simulink model "FOC_Modified"  (R2016b)
settings: Solver=FixedStepDiscrete  StartTime=0.0  StopTime=10.0  RelTol=1e-3  EnableMultiTasking=on
PreLoadFcn:
  | hdlcoderFocCurrentFixptHdlData
undefined symbols (not defined in the file): dataRange, paramCurrentControlSatVoltage
libraries: simulink x3
settings Model: Creator=mcorless  LastModifiedBy=paul.rogers
settings DataIOCC: LimitDataPoints=on  SaveFormat=Array
settings OptimizationCC: BlockReduction=off  ConditionallyExecuteInputs=off  DefaultParameterBehavior=Inlined  InlineInvariantSignals=on  LifeSpan=1
settings DebuggingCC: ArtificialAlgebraicLoopMsg=error  SolverPrmCheckMsg=warning  InheritedTsInSrcMsg=none  SingleTaskRateTransMsg=error  ParameterPrecisionLossMsg=none  SFUnexpectedBacktrackingDiag=warning  SFNoUnconditionalDefaultTransitionDiag=warning  SFExecutionAtInitializationDiag=none
settings HardwareCC: ProdBitPerPointer=32  ProdBitPerSizeT=32  ProdBitPerPtrDiffT=32  ProdLargestAtomicFloat=None  ProdIntDivRoundTo=Undefined  ProdEndianess=Unspecified  ProdWordSize=32  ProdHWDeviceType=ASIC/FPGA  ProdEqTarget=off
settings ModelReferenceCC: PropagateSignalLabelsOutOfModel=off
settings GRTTargetCC: TargetLangStandard=C89/C90 (ANSI)  GeneratePreprocessorConditionals=Disable all
settings ConfigComp: CovMetricSettings=dw  CovHtmlReporting=on  CovSaveCumulativeToWorkspaceVar=on  CovSaveSingleToWorkspaceVar=on  CovExternalEMLEnable=off  CovSFcnEnable=off

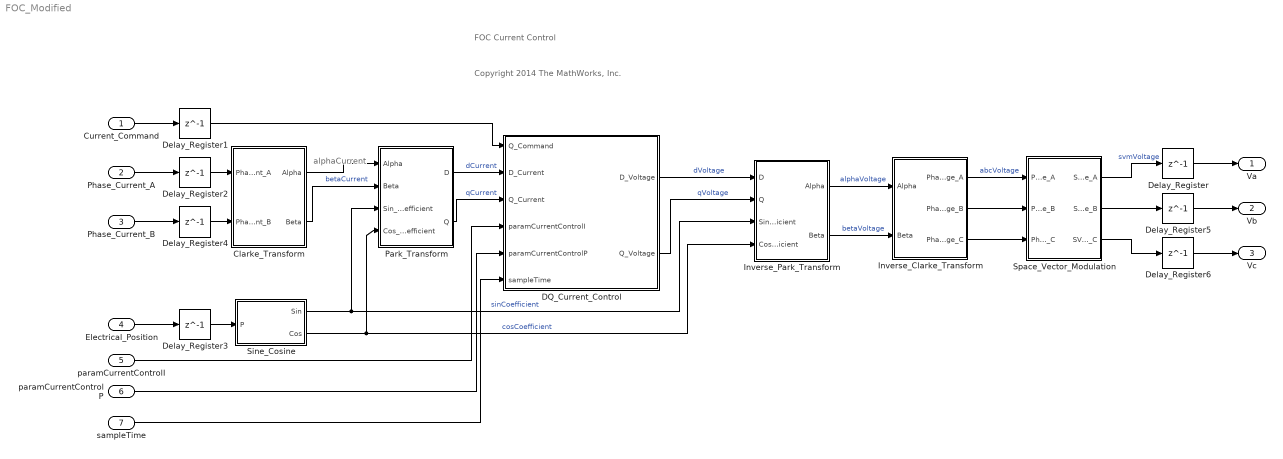
== system FOC_Modified ==
  note: alphaCurrent
  note: FOC Current Control
  note: Copyright 2014 The MathWorks, Inc.
  Current_Command : Inport  OutMin=dataRange.PhaseCurrent.Min  OutMax=dataRange.PhaseCurrent.Max  OutDataTypeStr=fixdt(1,16,12)  SampleTime=0.000000081
  Phase_Current_A : Inport  Port=2  OutMin=dataRange.PhaseCurrent.Min  OutMax=dataRange.PhaseCurrent.Max  OutDataTypeStr=fixdt(1,16,12)  SampleTime=0.000000081
  Phase_Current_B : Inport  Port=3  OutMin=dataRange.PhaseCurrent.Min  OutMax=dataRange.PhaseCurrent.Max  OutDataTypeStr=fixdt(1,16,12)  SampleTime=0.000000081
  Electrical_Position : Inport  Port=4  OutMin=0  OutMax=2*pi  OutDataTypeStr=fixdt(1,16,12)  SampleTime=0.000000081
  paramCurrentControlI : Inport  Port=5  OutDataTypeStr=fixdt(1,16,3)  SampleTime=0.000000081
  paramCurrentControlP : Inport  Port=6  OutDataTypeStr=fixdt(1,16,8)  SampleTime=0.000000081
  sampleTime : Inport  Port=7  OutDataTypeStr=fixdt(1,16,30)  SampleTime=0.000000081
  Clarke_Transform : Subsystem
      mask Display:
      | port_label('input',1,'ABC')
      | port_label('output',1,'\alpha','texmode', 'on')
      | port_label('output',2,'\beta','texmode', 'on')
  DQ_Current_Control : Subsystem
  Delay_Register{,1..6} (7 alike) : Delay  DelayLength=1
  Inverse_Clarke_Transform : Subsystem  VariantControl=INVERSE_CLARKE_TRANSFORM
      mask Display:
      | port_label('input',1,'\alpha','texmode', 'on')
      | port_label('input',2,'\beta','texmode', 'on')
      | port_label('output',1,'ABC')
  Inverse_Park_Transform : Subsystem
      mask Display:
      | port_label('input',1,'D')
      | port_label('input',2,'Q')
      | port_label('input',3,'Sin')
      | port_label('input',4,'Cos')
      | port_label('output',1,'\alpha','texmode', 'on')
      | port_label('output',2,'\beta','texmode', 'on')
  Park_Transform : Subsystem
      mask Display:
      | port_label('input',1,'\alpha','texmode', 'on')
      | port_label('input',2,'\beta','texmode', 'on')
      | port_label('input',3,'Sin')
      | port_label('input',4,'Cos')
      | port_label('output',1,'D')
      | port_label('output',2,'Q')
  Sine_Cosine : Subsystem
  Space_Vector_Modulation : Subsystem  VariantControl=SpaceVectorModulation_JB
      mask Display:
      | plot([0.000 0.020 0.041 0.061 0.082 0.102 0.122 0.143 0.163 0.184 0.204 0.224 0.245 0.265 0.286 0.306 0.327 0.347 0.367 0.388 0.408 0.429 0.449 0.469 0.490 0.510 0.531 0.551 0.571 0.592 0.612 0.633 0.653 0.673 0.694 0.714 0.735 0.755 0.776 0.796 0.816 0.837 0.857 0.878 0.898 0.918 0.939 0.959 0.980 1.000 ], ...
      |      [0.500 0.586 0.671 0.753 0.831 0.858 0.875 0.885 0.890 0.887 0.879 0.864 0.844 0.855 0.872 0.884 0.889 0.888 0.881 0.867 0.847 0.793 0.713 0.629 0.543 0.457 0.371 0.287 0.207 0.153 0.133 0.119 0.112 0.111 0.116 0.128 0.145 0.156 0.136 0.121 0.113 0.110 0.115 0.125 0.142 0.169 0.247 0.329 0.414 0.500 ])
  Va : Outport
  Vb : Outport  Port=2
  Vc : Outport  Port=3
  wires:
  Sine_Cosine/1(Sin) -> Park_Transform/3(Sin_Coefficient), Inverse_Park_Transform/3(Sin_Coefficient)  "sinCoefficient"
  Sine_Cosine/2(Cos) -> Park_Transform/4(Cos_Coefficient), Inverse_Park_Transform/4(Cos_Coefficient)  "cosCoefficient"
  Inverse_Clarke_Transform/1(Phase_Voltage_A) -> Space_Vector_Modulation/1(Phase_Voltage_A)  "abcVoltage"
  Electrical_Position/1 -> Delay_Register3/1
  Phase_Current_A/1 -> Delay_Register2/1
  Clarke_Transform/1(Alpha) -> Park_Transform/1(Alpha)
  Clarke_Transform/2(Beta) -> Park_Transform/2(Beta)  "betaCurrent"
  Inverse_Park_Transform/1(Alpha) -> Inverse_Clarke_Transform/1(Alpha)  "alphaVoltage"
  Inverse_Park_Transform/2(Beta) -> Inverse_Clarke_Transform/2(Beta)  "betaVoltage"
  Park_Transform/1(D) -> DQ_Current_Control/2(D_Current)  "dCurrent"
  Park_Transform/2(Q) -> DQ_Current_Control/3(Q_Current)  "qCurrent"
  Current_Command/1 -> Delay_Register1/1
  DQ_Current_Control/1(D_Voltage) -> Inverse_Park_Transform/1(D)  "dVoltage"
  DQ_Current_Control/2(Q_Voltage) -> Inverse_Park_Transform/2(Q)  "qVoltage"
  Delay_Register1/1 -> DQ_Current_Control/1(Q_Command)
  Delay_Register2/1 -> Clarke_Transform/1(Phase_Current_A)
  Delay_Register3/1 -> Sine_Cosine/1(P)
  paramCurrentControlI/1 -> DQ_Current_Control/4(paramCurrentControlI)
  paramCurrentControlP/1 -> DQ_Current_Control/5(paramCurrentControlP)
  sampleTime/1 -> DQ_Current_Control/6(sampleTime)
  Phase_Current_B/1 -> Delay_Register4/1
  Delay_Register4/1 -> Clarke_Transform/2(Phase_Current_B)
  Inverse_Clarke_Transform/2(Phase_Voltage_B) -> Space_Vector_Modulation/2(Phase_Voltage_B)
  Inverse_Clarke_Transform/3(Phase_Voltage_C) -> Space_Vector_Modulation/3(Phase_Voltage_C)
  Space_Vector_Modulation/2(SVM_Phase_Voltage_B) -> Delay_Register5/1
  Space_Vector_Modulation/1(SVM_Phase_Voltage_A) -> Delay_Register/1  "svmVoltage"
  Space_Vector_Modulation/3(SVM_Phase_Voltage_C) -> Delay_Register6/1
  Delay_Register5/1 -> Vb/1
  Delay_Register6/1 -> Vc/1
  Delay_Register/1 -> Va/1

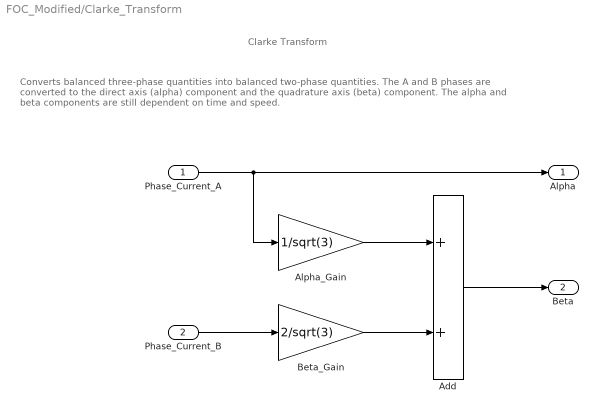
== system FOC_Modified/Clarke_Transform ==
  note: Clarke Transform
  note: Converts balanced three-phase quantities into balanced two-phase quantities.
      | The A and B phases are converted to the direct axis (alpha) component and the quadrature axis (beta) component.
      | The alpha and beta components are still dependent on time and speed.
  Phase_Current_A : Inport
  Phase_Current_B : Inport  Port=2
  Add : Sum  OutDataTypeStr=fixdt(1,16,11)
  Alpha_Gain : Gain  Gain=1/sqrt(3)  ParamDataTypeStr=fixdt(1,16,15)  OutDataTypeStr=fixdt(1,32,29)
  Beta_Gain : Gain  Gain=2/sqrt(3)  ParamDataTypeStr=fixdt(1,16,14)  OutDataTypeStr=fixdt(1,32,28)
  Alpha : Outport
  Beta : Outport  Port=2
  wires:
  Add/1 -> Beta/1
  Phase_Current_B/1 -> Beta_Gain/1
  Beta_Gain/1 -> Add/2
  Alpha_Gain/1 -> Add/1
  Phase_Current_A/1 -> Alpha_Gain/1, Alpha/1

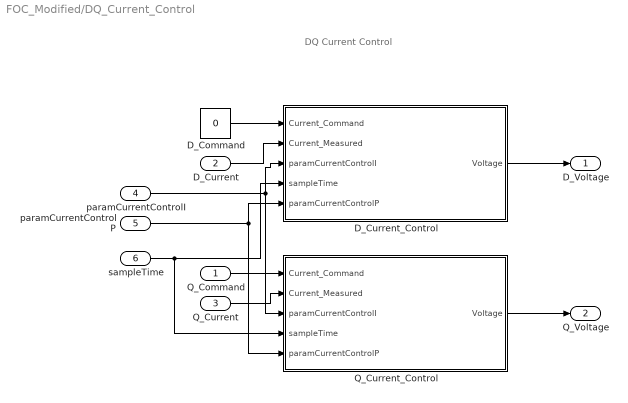
== system FOC_Modified/DQ_Current_Control ==
  note: DQ Current Control
  Q_Command : Inport  SampleTime=0.000000081
  D_Current : Inport  Port=2
  Q_Current : Inport  Port=3
  paramCurrentControlI : Inport  Port=4  SampleTime=0.000000081
  paramCurrentControlP : Inport  Port=5
  sampleTime : Inport  Port=6  SampleTime=0.000000081
  D_Command : Constant  Value=0  OutDataTypeStr=fixdt(1,16,12)  SampleTime=0.000000081
  D_Current_Control : Subsystem  TreatAsAtomicUnit=on
  Q_Current_Control : Subsystem  TreatAsAtomicUnit=on
  D_Voltage : Outport
  Q_Voltage : Outport  Port=2
  wires:
  Q_Current_Control/1(Voltage) -> Q_Voltage/1
  D_Current_Control/1(Voltage) -> D_Voltage/1
  D_Command/1 -> D_Current_Control/1(Current_Command)
  Q_Command/1 -> Q_Current_Control/1(Current_Command)
  Q_Current/1 -> Q_Current_Control/2(Current_Measured)
  D_Current/1 -> D_Current_Control/2(Current_Measured)
  sampleTime/1 -> D_Current_Control/4(sampleTime), Q_Current_Control/4(sampleTime)
  paramCurrentControlI/1 -> D_Current_Control/3(paramCurrentControlI), Q_Current_Control/3(paramCurrentControlI)
  paramCurrentControlP/1 -> D_Current_Control/5(paramCurrentControlP), Q_Current_Control/5(paramCurrentControlP)

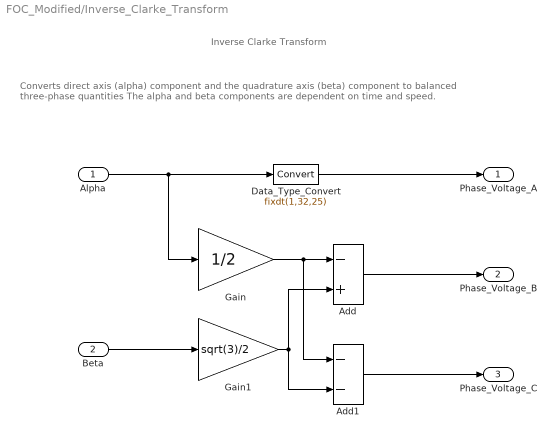
== system FOC_Modified/Inverse_Clarke_Transform ==
  note: Inverse Clarke Transform
  note: Converts direct axis (alpha) component and the quadrature axis (beta) component to balanced three-phase quantities
      | The alpha and beta components are dependent on time and speed.
  Alpha : Inport
  Beta : Inport  Port=2
  Add : Sum  Inputs=-+  OutDataTypeStr=fixdt(1,32,25)
  Add1 : Sum  Inputs=--  OutDataTypeStr=fixdt(1,32,25)
  Data_Type_Convert : DataTypeConversion  OutDataTypeStr=fixdt(1,32,25)  RndMeth=Simplest
  Gain : Gain  Gain=1/2  ParamDataTypeStr=fixdt(1,16,15)  OutDataTypeStr=fixdt(1,32,27)
  Gain1 : Gain  Gain=sqrt(3)/2  ParamDataTypeStr=fixdt(1,16,15)  OutDataTypeStr=fixdt(1,32,26)
  Phase_Voltage_A : Outport
  Phase_Voltage_B : Outport  Port=2
  Phase_Voltage_C : Outport  Port=3
  wires:
  Gain/1 -> Add1/1, Add/1
  Gain1/1 -> Add1/2, Add/2
  Add/1 -> Phase_Voltage_B/1
  Add1/1 -> Phase_Voltage_C/1
  Beta/1 -> Gain1/1
  Alpha/1 -> Gain/1, Data_Type_Convert/1
  Data_Type_Convert/1 -> Phase_Voltage_A/1

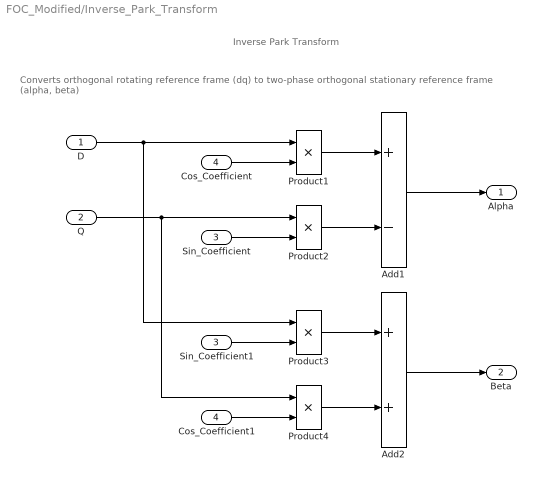
== system FOC_Modified/Inverse_Park_Transform ==
  note: Inverse Park Transform
  note: Converts orthogonal rotating reference frame (dq) to two-phase orthogonal stationary reference frame (alpha, beta)
  D : Inport
  Q : Inport  Port=2
  Sin_Coefficient : Inport  Port=3
  Cos_Coefficient : Inport  Port=4
  Add1 : Sum  Inputs=+-  OutDataTypeStr=fixdt(1,16,10)
  Add2 : Sum  OutDataTypeStr=fixdt(1,16,10)
  Cos_Coefficient1 : InportShadow  Port=4
  Product{1..4} (4 alike) : Product  OutDataTypeStr=fixdt(1,32,27)  RndMeth=Simplest
  Sin_Coefficient1 : InportShadow  Port=3
  Alpha : Outport
  Beta : Outport  Port=2
  wires:
  Add2/1 -> Beta/1
  Add1/1 -> Alpha/1
  Product3/1 -> Add2/1
  Product4/1 -> Add2/2
  Product1/1 -> Add1/1
  Product2/1 -> Add1/2
  Cos_Coefficient1/1 -> Product4/2
  Sin_Coefficient/1 -> Product2/2
  D/1 -> Product3/1, Product1/1
  Q/1 -> Product2/1, Product4/1
  Sin_Coefficient1/1 -> Product3/2
  Cos_Coefficient/1 -> Product1/2

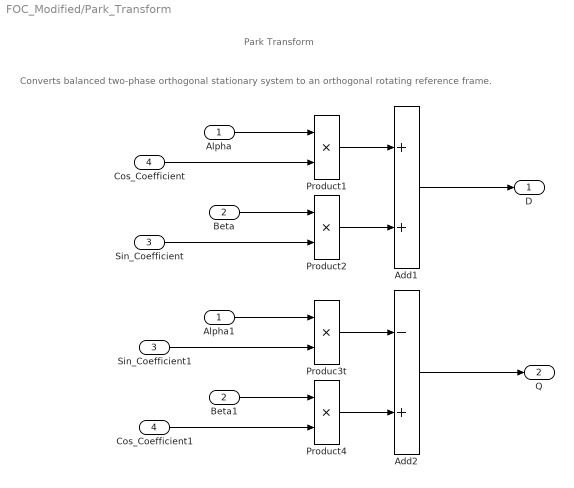
== system FOC_Modified/Park_Transform ==
  note: Park Transform
  note: Converts balanced two-phase orthogonal stationary system to an orthogonal rotating reference frame.
  Alpha : Inport
  Beta : Inport  Port=2
  Sin_Coefficient : Inport  Port=3
  Cos_Coefficient : Inport  Port=4
  Add1 : Sum  OutDataTypeStr=fixdt(1,32,27)
  Add2 : Sum  Inputs=-+  OutDataTypeStr=fixdt(1,32,27)
  Alpha1 : InportShadow
  Beta1 : InportShadow  Port=2
  Cos_Coefficient1 : InportShadow  Port=4
  Produc3t : Product  OutDataTypeStr=fixdt(1,32,28)  RndMeth=Simplest
  Product1 : Product  OutDataTypeStr=fixdt(1,32,28)  RndMeth=Simplest
  Product2 : Product  OutDataTypeStr=fixdt(1,32,27)  RndMeth=Simplest
  Product4 : Product  OutDataTypeStr=fixdt(1,32,27)  RndMeth=Simplest
  Sin_Coefficient1 : InportShadow  Port=3
  D : Outport
  Q : Outport  Port=2
  wires:
  Produc3t/1 -> Add2/1
  Product4/1 -> Add2/2
  Product1/1 -> Add1/1
  Product2/1 -> Add1/2
  Alpha1/1 -> Produc3t/1
  Sin_Coefficient1/1 -> Produc3t/2
  Cos_Coefficient1/1 -> Product4/2
  Beta1/1 -> Product4/1
  Alpha/1 -> Product1/1
  Cos_Coefficient/1 -> Product1/2
  Beta/1 -> Product2/1
  Sin_Coefficient/1 -> Product2/2
  Add1/1 -> D/1
  Add2/1 -> Q/1

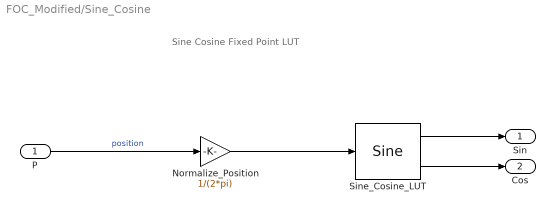
== system FOC_Modified/Sine_Cosine ==
  note: Sine Cosine Fixed Point LUT
  P : Inport
  Normalize_Position : Gain  Gain=1/(2*pi)  ParamDataTypeStr=fixdt(1,16,17)  OutMin=0  OutMax=1  OutDataTypeStr=fixdt(1,32,30)
      settings: AttributesFormatString=|
      | ------------------------------
      | Gain = %<Gain>
  Sine_Cosine_LUT : simulink/Lookup Tables/Sine  Formula=sin(2*pi*u) and cos(2*pi*u)  NumDataPoints=(2^5)+1  OutputWordLength=16  InternalRulePriority=Speed
  Sin : Outport
  Cos : Outport  Port=2
  wires:
  Sine_Cosine_LUT/2 -> Cos/1
  Sine_Cosine_LUT/1 -> Sin/1
  Normalize_Position/1 -> Sine_Cosine_LUT/1
  P/1 -> Normalize_Position/1  "position"

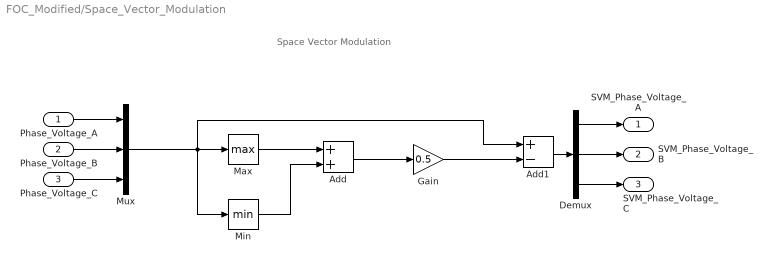
== system FOC_Modified/Space_Vector_Modulation ==
  note: Space Vector Modulation
  Phase_Voltage_A : Inport
  Phase_Voltage_B : Inport  Port=2
  Phase_Voltage_C : Inport  Port=3
  Add : Sum  OutDataTypeStr=fixdt(1,16,8)
  Add1 : Sum  Inputs=+-  OutDataTypeStr=fixdt(1,16,8)
  Demux : Demux  Outputs=3
  Gain : Gain  Gain=0.5  ParamDataTypeStr=fixdt(1,16,15)  OutDataTypeStr=fixdt(1,32,25)
  Max : MinMax  Function=max
  Min : MinMax
  Mux : Mux  Inputs=3
  SVM_Phase_Voltage_A : Outport
  SVM_Phase_Voltage_B : Outport  Port=2
  SVM_Phase_Voltage_C : Outport  Port=3
  wires:
  Add/1 -> Gain/1
  Max/1 -> Add/1
  Min/1 -> Add/2
  Gain/1 -> Add1/2
  Phase_Voltage_C/1 -> Mux/3
  Phase_Voltage_B/1 -> Mux/2
  Phase_Voltage_A/1 -> Mux/1
  Mux/1 -> Add1/1, Min/1, Max/1
  Add1/1 -> Demux/1
  Demux/3 -> SVM_Phase_Voltage_C/1
  Demux/2 -> SVM_Phase_Voltage_B/1
  Demux/1 -> SVM_Phase_Voltage_A/1

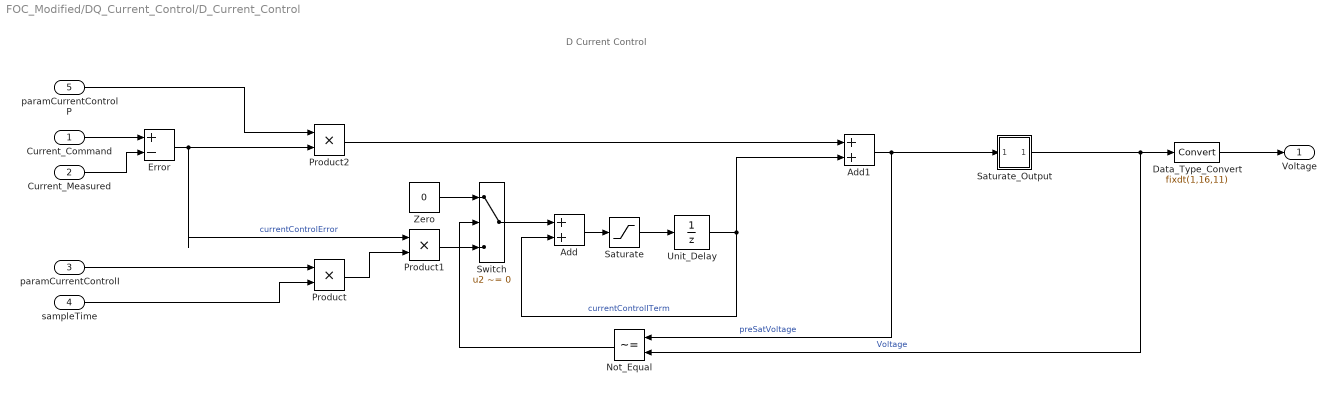
== system FOC_Modified/DQ_Current_Control/D_Current_Control ==
  note: D Current Control
  Current_Command : Inport
  Current_Measured : Inport  Port=2
  paramCurrentControlI : Inport  Port=3
  sampleTime : Inport  Port=4
  paramCurrentControlP : Inport  Port=5
  Add : Sum  OutDataTypeStr=fixdt(1,32,27)
  Add1 : Sum  OutDataTypeStr=fixdt(1,32,20)
  Data_Type_Convert : DataTypeConversion  OutDataTypeStr=fixdt(1,16,11)  RndMeth=Simplest
  Error : Sum  Inputs=+-  OutDataTypeStr=fixdt(1,16,11)
  Not_Equal : RelationalOperator  Operator=~=  OutDataTypeStr=boolean  RndMeth=Nearest
  Product : Product  OutDataTypeStr=fixdt(1,16,19)
  Product1 : Product  OutDataTypeStr=fixdt(1,32,31)
  Product2 : Product
  Saturate : Saturate  UpperLimit=dataRange.DqVoltage.Max  LowerLimit=dataRange.DqVoltage.Min
      settings: AttributesFormatString=|
      | --------------------------------------------
      | Upper = %<UpperLimit>
      | Lower = %<LowerLimit>
  Saturate_Output : Subsystem  mask(Saturate Magnitude){magnitudeLimit=paramCurrentControlSatVoltage}
      mask prompts: magnitudeLimit "Magnitude limit:"
      mask help:
      | Saturates input where:
      |    Upper limit =   Magnitude limit
      |    Lower limit = - Magnitude limit
      settings: AttributesFormatString=|
      | --------------------------------------------
      | Upper limit = %<magnitudeLimit>
      | Lower limit = -%<magnitudeLimit>
      mask Display: plot([0.15 0.85],[.5 .5],[.5 .5],[0.05 0.95],0.15+0.7*[0 .25 .75 1],0.05+0.9*[.25 .25 .75 .75]);
  Switch : Switch  Criteria=u2 ~= 0  OutDataTypeStr=fixdt(1,32,31)
  Unit_Delay : UnitDelay  SampleTime=-1
  Zero : Constant  Value=0  OutDataTypeStr=fixdt(1,16,0)  SampleTime=0.000000081
  Voltage : Outport
  wires:
  Data_Type_Convert/1 -> Voltage/1
  Product1/1 -> Switch/3
  Product/1 -> Product1/2
  sampleTime/1 -> Product/2
  paramCurrentControlI/1 -> Product/1
  Saturate/1 -> Unit_Delay/1
  Zero/1 -> Switch/1
  Switch/1 -> Add/1
  Not_Equal/1 -> Switch/2
  Add/1 -> Saturate/1
  Saturate_Output/1(Out) -> Data_Type_Convert/1, Not_Equal/2  "Voltage"
  Error/1 -> Product2/2, Product1/1  "currentControlError"
  Current_Command/1 -> Error/1
  Add1/1 -> Saturate_Output/1(In), Not_Equal/1  "preSatVoltage"
  Unit_Delay/1 -> Add1/2, Add/2  "currentControlITerm"
  Current_Measured/1 -> Error/2
  Product2/1 -> Add1/1
  paramCurrentControlP/1 -> Product2/1

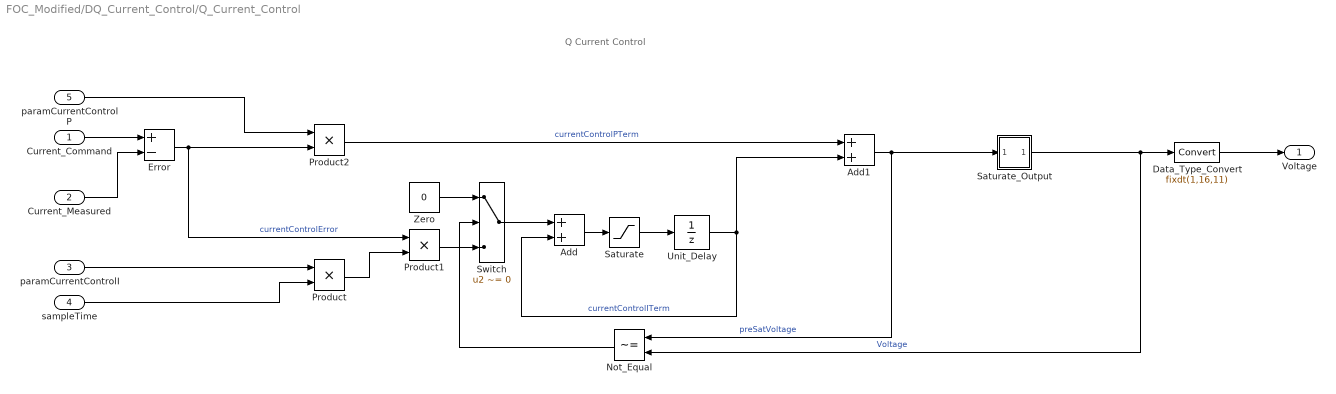
== system FOC_Modified/DQ_Current_Control/Q_Current_Control ==
  note: Q Current Control
  Current_Command : Inport
  Current_Measured : Inport  Port=2
  paramCurrentControlI : Inport  Port=3
  sampleTime : Inport  Port=4
  paramCurrentControlP : Inport  Port=5
  Add : Sum  OutDataTypeStr=fixdt(1,32,27)
  Add1 : Sum  OutDataTypeStr=fixdt(1,32,20)
  Data_Type_Convert : DataTypeConversion  OutDataTypeStr=fixdt(1,16,11)  RndMeth=Simplest
  Error : Sum  Inputs=+-  OutDataTypeStr=fixdt(1,16,11)
  Not_Equal : RelationalOperator  Operator=~=  OutDataTypeStr=boolean  RndMeth=Nearest
  Product : Product  OutDataTypeStr=fixdt(1,16,19)
  Product1 : Product  OutDataTypeStr=fixdt(1,32,31)
  Product2 : Product
  Saturate : Saturate  UpperLimit=dataRange.DqVoltage.Max  LowerLimit=dataRange.DqVoltage.Min
      settings: AttributesFormatString=|
      | --------------------------------------------
      | Upper = %<UpperLimit>
      | Lower = %<LowerLimit>
  Saturate_Output : Subsystem  mask(Saturate Magnitude){magnitudeLimit=paramCurrentControlSatVoltage}
      mask prompts: magnitudeLimit "Magnitude limit:"
      mask help:
      | Saturates input where:
      |    Upper limit =   Magnitude limit
      |    Lower limit = - Magnitude limit
      settings: AttributesFormatString=|
      | --------------------------------------------
      | Upper limit = %<magnitudeLimit>
      | Lower limit = -%<magnitudeLimit>
      mask Display: plot([0.15 0.85],[.5 .5],[.5 .5],[0.05 0.95],0.15+0.7*[0 .25 .75 1],0.05+0.9*[.25 .25 .75 .75]);
  Switch : Switch  Criteria=u2 ~= 0  OutDataTypeStr=fixdt(1,32,31)
  Unit_Delay : UnitDelay  SampleTime=-1
  Zero : Constant  Value=0  OutDataTypeStr=fixdt(1,16,0)  SampleTime=0.000000081
  Voltage : Outport
  wires:
  Current_Measured/1 -> Error/2
  Unit_Delay/1 -> Add/2, Add1/2  "currentControlITerm"
  Add1/1 -> Not_Equal/1, Saturate_Output/1(In)  "preSatVoltage"
  Current_Command/1 -> Error/1
  Product2/1 -> Add1/1  "currentControlPTerm"
  Error/1 -> Product2/2, Product1/1  "currentControlError"
  Saturate_Output/1(Out) -> Not_Equal/2, Data_Type_Convert/1  "Voltage"
  Add/1 -> Saturate/1
  Not_Equal/1 -> Switch/2
  Switch/1 -> Add/1
  Zero/1 -> Switch/1
  Saturate/1 -> Unit_Delay/1
  paramCurrentControlI/1 -> Product/1
  sampleTime/1 -> Product/2
  Product/1 -> Product1/2
  Product1/1 -> Switch/3
  Data_Type_Convert/1 -> Voltage/1
  paramCurrentControlP/1 -> Product2/1

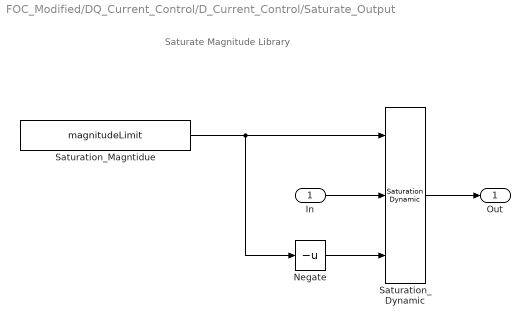
== system FOC_Modified/DQ_Current_Control/D_Current_Control/Saturate_Output ==
  note: Saturate Magnitude Library
  In : Inport
  Negate : UnaryMinus  SampleTime=0.000000081
  Saturation_Dynamic : simulink/Discontinuities/Saturation Dynamic  OutMin=[]  OutMax=[]  OutDataTypeStr=Inherit: Same as second input  OutDataType=fixdt(1, 16)  OutScaling=2^-10  DoSatur=off
  Saturation_Magntidue : Constant  Value=magnitudeLimit  OutDataTypeStr=fixdt(1,16,11)  SampleTime=0.000000081
  Out : Outport
  wires:
  Saturation_Magntidue/1 -> Negate/1, Saturation_Dynamic/1
  Saturation_Dynamic/1 -> Out/1
  Negate/1 -> Saturation_Dynamic/3
  In/1 -> Saturation_Dynamic/2

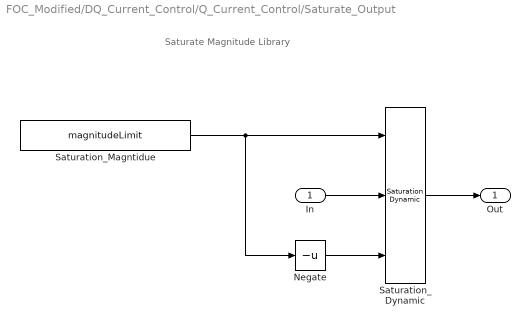
== system FOC_Modified/DQ_Current_Control/Q_Current_Control/Saturate_Output ==
  note: Saturate Magnitude Library
  In : Inport
  Negate : UnaryMinus  SampleTime=0.000000081
  Saturation_Dynamic : simulink/Discontinuities/Saturation Dynamic  OutMin=[]  OutMax=[]  OutDataTypeStr=Inherit: Same as second input  OutDataType=fixdt(1, 16)  OutScaling=2^-10  DoSatur=off
  Saturation_Magntidue : Constant  Value=magnitudeLimit  OutDataTypeStr=fixdt(1,16,11)  SampleTime=0.000000081
  Out : Outport
  wires:
  In/1 -> Saturation_Dynamic/2
  Negate/1 -> Saturation_Dynamic/3
  Saturation_Dynamic/1 -> Out/1
  Saturation_Magntidue/1 -> Saturation_Dynamic/1, Negate/1
